simulink model "Foc_model_Matlab_ultimo"  (R2024b)
settings: Solver=FixedStepDiscrete  StartTime=0.0  StopTime=7  FixedStep=Ts_simulink  RelTol=1e-3  EnableMultiTasking=on
PreLoadFcn:
  | mcb_pmsm_foc_hall_S32K144EVB_data;
InitFcn:
  | mbd_s32k_consistency_checks(bdroot(gcs));
model workspace (MAT data in the model file):
  IDC_OVERCURRENT : Simulink.Parameter (value not decoded)
  VDC_OVERVOLTAGE : Simulink.Parameter (value not decoded)
  VDC_UNDERVOLTAGE : Simulink.Parameter (value not decoded)
undefined symbols (not defined in the file or in its folder): DiscIntNeverNeededParam, epsilon, External, inverter, Kcd, Kcq, Kcs, Kid, Kiq, lambda, LQFP, mcb_isCodeGenVar, mcb_isSimVar, One, PI_params, pmsm, PU_System, rho, Shot, sigbuilder_block, TRGMUX_PDB_TRIG, Ts, Ts_motor, Ts_simulink, Ts_speed
libraries: mbd_s32k1xx_ec_toolbox x39, mcbcontrolslib x9, simulink x7, mcbpositiondecoderlib x6, mbd_msd_ec_toolbox x5, hdlsllib x4, slpidlib x3, mcbhdlpositiondecoderlib x1, mcbplantlib x1, autolibpmsmexterior x1
(part 3 of 3)

== system Foc_model_Matlab_ultimo/CurrentControl/Input Scaling/Read_Sensor (sim)/Subsystem ==
  Pos_Sim : Inport
  IIR Filter : mcbcontrolslib/IIR Filter  Commented=through  VariantControl=Low Pass Filter  VariantSelect=Low-pass  FilterConstantInputType=Specify via dialog  Filter_constant=0.01  advancedSettings=off  Ts=50e-6  cutOff_freq=32.1525
  Mechanical to Electrical Position : mcbpositiondecoderlib/Mechanical to Electrical Position  PolePairsInputType=Specify via dialog  NrPP=pmsm.p  selectedRange=Per unit  MechOfstInputType=Specify via dialog  mechOffsetIn=0  maxAngleIn=1  InputDataType=dataType  VariantSelect=floating-point
  Speed Measurement : mcbpositiondecoderlib/Speed Measurement  PositionUnit=Per unit  PositionScalingDatatype=uint32  SpeedCalculationMode=Time interval for speed calculation  SampleTimeAsync=Ts  MaximumApplicationSpeed=6000  SpeedResolution=5e-6  DelayLength=10  MaximumMeasurableSpeed=29999  MeasurableSpeedResolution=1.397e-05  SpeedUnit=Per unit based on dialog  PerUnitSpeed=pmsm.N_max  SpeedDataType=single
  Theta : Outport
  Speed : Outport  Port=2
  wires:
  Mechanical to Electrical Position/1 -> Theta/1
  Speed Measurement/1 -> IIR Filter/1
  Pos_Sim/1 -> Mechanical to Electrical Position/1, Speed Measurement/1
  IIR Filter/1 -> Speed/1

== system Foc_model_Matlab_ultimo/HallCodeGen/Subsystem2/ADC1_IRQHandler/FaultDetection ==
  Vdc : Inport
  Idc : Inport  Port=2
  ADC1_AD7_Offset : Constant  Value=17  OutDataTypeStr=single
  ADC_AD6 offset and Logic power supply compensation : Constant  Value=2090  OutDataTypeStr=single
  Abs : Abs  SaturateOnIntegerOverflow=off
  Add : Sum  Inputs=-+  OutMin=0  OutMax=4095  OutDataTypeStr=single  AccumDataTypeStr=single  InputSameDT=on
  Check_Voltage_Current_Limits : If  NumInputs=2  IfExpression=(u1 < VDC_UNDERVOLTAGE) | (u1 > VDC_OVERVOLTAGE) | (u2 > IDC_OVERCURRENT)  ShowElse=off
  Data Type Conversion : DataTypeConversion  OutDataTypeStr=single  SaturateOnIntegerOverflow=off  RndMeth=Floor
  Data Type Conversion1 : DataTypeConversion  OutDataTypeStr=single  SaturateOnIntegerOverflow=off  RndMeth=Floor
  FAILURE : Subsystem  TreatAsAtomicUnit=on
  Product : Product  OutDataTypeStr=single
  Product1 : Product  OutDataTypeStr=single
  Sum : Sum  Inputs=+-  OutDataTypeStr=single  AccumDataTypeStr=single
  bits2amps : Constant  Value=16.5/2048  OutDataTypeStr=single
  bits2volts : Constant  Value=45/4095  OutDataTypeStr=single
  wires:
  Check_Voltage_Current_Limits/1 -> FAILURE/Action
  Idc/1 -> Data Type Conversion/1
  Data Type Conversion/1 -> Abs/1
  Vdc/1 -> Data Type Conversion1/1
  Abs/1 -> Sum/1
  ADC_AD6 offset and Logic power supply compensation/1 -> Sum/2
  Sum/1 -> Product/1  "Idc_afterOffset"
  Product/1 -> Check_Voltage_Current_Limits/2
  bits2amps/1 -> Product/2
  ADC1_AD7_Offset/1 -> Add/1
  Data Type Conversion1/1 -> Add/2
  bits2volts/1 -> Product1/2
  Add/1 -> Product1/1
  Product1/1 -> Check_Voltage_Current_Limits/1

== system Foc_model_Matlab_ultimo/CurrentControl/Input Scaling/Read_Sensor (codegen)/Calculate Position from Hall/Atomic Hall Reading ==
  Data Store Read2 : DataStoreRead  DataStoreName=GlobalSpeedCount  IndexOptions=Index vector (dialog)  Indices=1  OutputSizes=1
  Data Store Read3 : DataStoreRead  DataStoreName=GlobalDirection  IndexOptions=Index vector (dialog)  Indices=1  OutputSizes=1
  Data Store Read4 : DataStoreRead  DataStoreName=GlobalSpeedValidity  IndexOptions=Index vector (dialog)  Indices=1  OutputSizes=1
  Data Store Read5 : DataStoreRead  Priority=1  DataStoreName=HallStateChangeFlag  IndexOptions=Index vector (dialog)  Indices=1  OutputSizes=1
  Hall Read : Subsystem
  Read_Register : mbd_s32k1xx_ec_toolbox/Utility Blocks/Read_Register  periph=ADC0  reg=SC1A  addr=0x4003B000  regSize=32  pcc_clock=ADC0_CLK
  HallState : Outport
  Count : Outport  Port=2
  SpeedCount : Outport  Port=3
  Dir : Outport  Port=4
  SpeedValidity : Outport  Port=5
  Hallchange : Outport  Port=6
  wires:
  Data Store Read4/1 -> SpeedValidity/1
  Data Store Read5/1 -> Hallchange/1
  Data Store Read2/1 -> SpeedCount/1
  Data Store Read3/1 -> Dir/1
  Hall Read/1(Out1) -> HallState/1
  Read_Register/1 -> Count/1

== system Foc_model_Matlab_ultimo/HallCodeGen/Subsystem2/ADC1_IRQHandler/FaultDetection/FAILURE ==
  Action Port : ActionPort  ActionPortLabel=if((u1 < VDC_UNDERVOLTAGE) | (u1 > VDC_OVERVOLTAGE) | (u2 > IDC_OVERCURRENT))
  FAULT_read : DataStoreRead  DataStoreName=FAULT  IndexOptions=Index vector (dialog)  Indices=1  OutputSizes=1
  Failed Subsystem : Subsystem  TreatAsAtomicUnit=on
  If : If  IfExpression=u1 == 0  ShowElse=off
  wires:
  If/1 -> Failed Subsystem/Action
  FAULT_read/1 -> If/1

== system Foc_model_Matlab_ultimo/CurrentControl/Input Scaling/Read_Sensor (codegen)/Calculate Position from Hall/Atomic Hall Reading/Hall Read ==
  Add1 : Sum  Inputs=+++  OutDataTypeStr=Inherit: Inherit via back propagation
  Bit Shift : hdlsllib/Logic and Bit Operations/Bit Shift  mode=Shift Left Logical  N=2
  Bit Shift1 : hdlsllib/Logic and Bit Operations/Bit Shift  mode=Shift Left Logical  N=1
  Data Type Conversion2 : DataTypeConversion  OutDataTypeStr=uint32  SaturateOnIntegerOverflow=off  RndMeth=Floor
  Data Type Conversion3 : DataTypeConversion  OutDataTypeStr=uint32  SaturateOnIntegerOverflow=off  RndMeth=Floor
  Data Type Conversion6 : DataTypeConversion  OutDataTypeStr=uint32  SaturateOnIntegerOverflow=off  RndMeth=Floor
  Digital_Input_HALL_A : mbd_s32k1xx_ec_toolbox/GPIO Blocks/Digital_Input  gpio_pin=PTD11: [PTD11 | Port D I/O]  pull_resistor=None  passive_filter=off
  Digital_Input_HALL_B : mbd_s32k1xx_ec_toolbox/GPIO Blocks/Digital_Input  gpio_pin=PTD10: [PTD10 | Port D I/O]  pull_resistor=None  passive_filter=off
  Digital_Input_HALL_C : mbd_s32k1xx_ec_toolbox/GPIO Blocks/Digital_Input  gpio_pin=PTA1: [PTA1 | Port A I/O]  pull_resistor=None  passive_filter=off
  Out1 : Outport
  wires:
  Add1/1 -> Out1/1
  Data Type Conversion2/1 -> Bit Shift1/1
  Bit Shift/1 -> Add1/1  "HALL_C_controller"
  Bit Shift1/1 -> Add1/2  "HALL_B_controller"
  Data Type Conversion6/1 -> Add1/3  "HALL_A_controller"
  Data Type Conversion3/1 -> Bit Shift/1
  Digital_Input_HALL_C/1 -> Data Type Conversion3/1
  Digital_Input_HALL_B/1 -> Data Type Conversion2/1
  Digital_Input_HALL_A/1 -> Data Type Conversion6/1

== system Foc_model_Matlab_ultimo/HallCodeGen/Subsystem2/ADC1_IRQHandler/FaultDetection/FAILURE/Failed Subsystem ==
  Action Port : ActionPort  ActionPortLabel=if(u1 == 0)
  FAULT_write : DataStoreWrite  DataStoreName=FAULT  IndexOptions=Index vector (dialog)  Indices=1  OutputSizes=1
  FTM_PWM_Disable_Enable : mbd_s32k1xx_ec_toolbox/Motor Control Blocks/FTM Blocks/FTM_PWM_Disable_Enable  Priority=1  ftmModule=3  action=Disable
  NOK : Constant  OutDataTypeStr=boolean
  TPP_Functional_Mode : mbd_msd_ec_toolbox/TPP/TPP_Functional_Mode  tppInstance=0  action=Sleep
  wires:
  NOK/1 -> FAULT_write/1

== stateflow chart Foc_model_Matlab_ultimo/Hardware Initialization/Enable PDB and start FTM ==
  settings: sampleTime=0.500
  state A
  state END
  (default) -> A
  A -> END : {enablePDB;}
  END -> END : {Normal_Op;}
  events: enablePDB output FUNCTION_CALL_EVENT; Normal_Op output FUNCTION_CALL_EVENT

== matlab function Foc_model_Matlab_ultimo/CurrentControl/Control_System/Current_Controllers/PI_Controller_Id/MATLAB Function1 ==
  data: error input; V_ref output; Kp input; Ki input; upper_limit input; lower_limit input; reset input
function V_ref = PI_controller(error, Kp, Ki, upper_limit, lower_limit, reset)
    % Variabili persistenti per memorizzare i valori precedenti
    persistent integral

    % Assicuro che tutte le variabili siano di tipo single
    error = single(error);
    Kp = single(Kp);
    Ki = single(Ki);
    upper_limit = single(upper_limit);
    lower_limit = single(lower_limit);
    reset = single(reset);

    % Inizializzo le variabili se sono vuote o se il reset è richiesto
    if isempty(integral) || reset
        integral = single(0);
    end

    % Calcolo il termine proporzionale
    P = Kp * error;

    % Aggiorno l'integrale solo se l'uscita non è saturata o se l'errore è in direzione di ridurre la saturazione
    if (P + Ki * integral < upper_limit && P + Ki * integral > lower_limit) || ...
       (P + Ki * integral >= upper_limit && error < 0) || ...
       (P + Ki * integral <= lower_limit && error > 0)
        integral = integral + error;
    end

    % Calcolo la tensione di riferimento
    V_ref_unsat = P + Ki * integral;

    % Applico la saturazione alla tensione di riferimento
    V_ref = min(max(V_ref_unsat, lower_limit), upper_limit);
    
end

== matlab function Foc_model_Matlab_ultimo/CurrentControl/Control_System/Current_Controllers/PI_Controller_Iq/MATLAB Function1 ==
  data: error input; V_ref output; Kp input; Ki input; upper_limit input; lower_limit input; reset input
function V_ref = PI_controller(error, Kp, Ki, upper_limit, lower_limit, reset)
    % Variabili persistenti per memorizzare i valori precedenti
    persistent integral

     % Assicuro che tutte le variabili siano di tipo single
    error = single(error);
    Kp = single(Kp);
    Ki = single(Ki);
    upper_limit = single(upper_limit);
    lower_limit = single(lower_limit);
    reset = single(reset);

    % Inizializzo le variabili se sono vuote o se il reset è richiesto
    if isempty(integral) || reset
        integral = single(0);
    end

    % Calcolo il termine proporzionale
    P = Kp * error;

    % Aggiorno l'integrale solo se l'uscita non è saturata o se l'errore è in direzione di ridurre la saturazione
    if (P + Ki * integral < upper_limit && P + Ki * integral > lower_limit) || ...
       (P + Ki * integral >= upper_limit && error < 0) || ...
       (P + Ki * integral <= lower_limit && error > 0)
        integral = integral + error;
    end

    % Calcolo la tensione di riferimento
    V_ref_unsat = P + Ki * integral;

    % Applico la saturazione alla tensione di riferimento
    V_ref = min(max(V_ref_unsat, lower_limit), upper_limit);
    
end

== matlab function Foc_model_Matlab_ultimo/SpeedControl/STSMC/MATLAB Function ==
  data: errore_velocita input; errore_posizione input; accelerazione_ref input; N_fb input; lambda input; epsilon input; rho input; J input; B input; Kt input; limit input; I_ref output; T_eq output; T_n output; s output
function [I_ref,T_eq, T_n, s] = SMC3(errore_velocita, errore_posizione, accelerazione_ref, N_fb, lambda, epsilon, rho, J, B, Kt, limit)

    % Inizializzazione variabili
    T_n = single(0);
    s = errore_velocita + lambda*errore_posizione;       % Superficie di scorrimento

    %sat(s)
    if abs(s) > epsilon
        T_n = - rho*sign(s);
    else
        T_n = - rho*(s/epsilon);
    end

    % Legge di controllo
    T_eq = B*N_fb + J*(accelerazione_ref+lambda*(errore_velocita));
    I_ref_unsat = (T_eq + T_n)/Kt;
   

    % Applico la saturazione alla corrente di riferimento
    I_ref = min(max(I_ref_unsat, - limit), limit);

== matlab function Foc_model_Matlab_ultimo/SpeedControl/STSMC/MATLAB Function1 ==
  data: N_ref input; N_fb input; lambda input; epsilon input; theta input; J input; B input; Kt input; limit input; I_ref output; reset input; T_eq output; T_n output; s output
function [I_ref,T_eq, T_n, s] = SMC2(N_ref, N_fb, lambda, epsilon, theta, J, B, Kt, limit, reset)
    % Variabili persistenti per memorizzare i valori precedenti
    persistent N_ref_pre
    persistent N_fb_pre
    persistent T_n_pre
    T_n = single(0);

    % Inizializzo le variabili se sono vuote o se il reset è richiesto
    if isempty(N_ref_pre) || reset
        N_ref_pre = single(0);
    end
    % Inizializzo le variabili se sono vuote o se il reset è richiesto
    if isempty(N_fb_pre) || reset
        N_fb_pre = single(0);
    end
    % Inizializzo le variabili se sono vuote o se il reset è richiesto
    if isempty(T_n_pre) || reset
        T_n_pre = single(0);
    end

    speed_error = N_fb - N_ref;
    speed_error_pre = N_fb_pre - N_ref_pre;

    s = speed_error + lambda*speed_error_pre;

    %sat(s)
    if abs(s) > epsilon
        T_n = -theta*sign(s);
    else
        T_n = -theta*(s/epsilon);
    end

    %control law
    T_eq = B*N_ref_pre + J*(N_ref-lambda*(speed_error));
    I_ref_unsat = (T_eq + T_n)/Kt;

    N_ref_pre = N_ref;
    N_fb_pre = N_fb;
    T_n_pre = T_n;
    

    % Applico la saturazione alla corrente di riferimento
    I_ref = min(max(I_ref_unsat, - limit), limit);

== matlab function Foc_model_Matlab_ultimo/CurrentControl/Control_System/Current_Controllers/PI_Controller_Id/MATLAB Function ==
  data: gamma1 input; Kcd output; Kidtd output; Rs input; Ld input
function [Kcd, Kidtd] = fcn(gamma1, Rs, Ld)
    zeta1 = 0.707;
    wnd = (1/(1-gamma1))*(Rs/Ld);
    Kcd = (2*zeta1*wnd*Ld)-Rs;
    t_id = (2*zeta1*wnd*Ld-Rs)/(wnd^2*Ld);
    Kid = Kcd/t_id;
    Kidtd = Kid*t_id;

== matlab function Foc_model_Matlab_ultimo/CurrentControl/Control_System/Current_Controllers/PI_Controller_Iq/MATLAB Function ==
  data: gamma1 input; Kcq output; Kiqtq output; Rs input; Lq input
function [Kcq, Kiqtq] = fcn(gamma1, Rs, Lq)
    zeta1 = 0.707;
    wnq = (1/(1-gamma1))*(Rs/Lq);
    Kcq = (2*zeta1*wnq*Lq)-Rs;
    t_iq = (2*zeta1*wnq*Lq-Rs)/(wnq^2*Lq);
    Kiq = Kcq/t_iq;
    Kiqtq = Kiq*t_iq;

== matlab function Foc_model_Matlab_ultimo/CurrentControl/STSMO/Back-EMF Estimation ==
  data: v_alpha input; di_alpha_est output; di_beta_est output; e_alpha output; e_beta output; v_beta input; sat_ia input; sat_ib input; int_sat_ia input; int_sat_ib input; i_alpha_err input; i_beta_err input; i_alpha_est input; i_beta_est input; K1 input; K2 input
function [di_alpha_est, di_beta_est, e_alpha, e_beta]   = fcn(v_alpha, v_beta, sat_ia, sat_ib, int_sat_ia, int_sat_ib, i_alpha_err, i_beta_err, i_alpha_est, i_beta_est, K1, K2)


k1 = K1;
k2 = K2;         
R = 0.6367; %pmsm.Rs;
L = 0.000375; %pmsm.Ld;

z_alpha = k1*sqrt(abs(i_alpha_err))*sat_ia + k2*int_sat_ia;
z_beta = k1*sqrt(abs(i_beta_err))*sat_ib + k2*int_sat_ib;

di_alpha_est = -(R/L)*i_alpha_est + (1/L)*v_alpha - (1/L)*z_alpha;
di_beta_est = -(R/L)*i_beta_est + (1/L)*v_beta - (1/L)*z_beta;

e_alpha = z_alpha;
e_beta = z_beta;

== matlab function Foc_model_Matlab_ultimo/CurrentControl/STSMO/Saturation  ==
  data: i_alpha input; sat_ia_error output; i_beta input; i_alpha_est input; i_beta_est input; sat_ib_error output; ia_error output; ib_error output; epsilona input; epsilonb input
function [sat_ia_error, sat_ib_error, ia_error, ib_error] = fcn( i_alpha, i_beta, i_alpha_est, i_beta_est, epsilona, epsilonb)

epsilon_a = epsilona;
epsilon_b = epsilonb;


ia_error = i_alpha_est - i_alpha;
ib_error = i_beta_est - i_beta;

if abs(ia_error) > epsilon_a
    sat_ia_error = sign(ia_error);
else
    sat_ia_error = abs(ia_error) / epsilon_a;
end

if abs(ib_error) > epsilon_b
    sat_ib_error = sign(ib_error);
else
    sat_ib_error = abs(ib_error) / epsilon_b;
end
